simulink model "controladorultimo"  (Simulink 7.9)
settings: Solver=ode45  StartTime=0.0  StopTime=100  RelTol=1e-3
settings Model: Creator=Miguel Faggioni  LastModifiedBy=Miguel Faggioni
settings DataIOCC: TimeSaveName=t

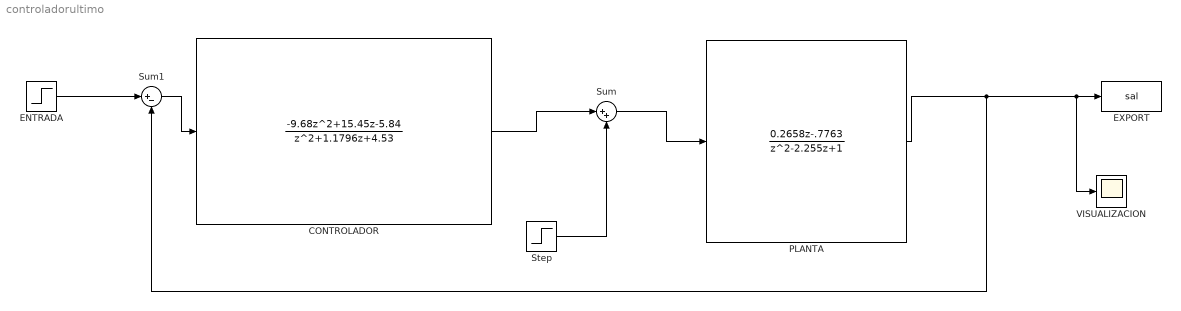
== system controladorultimo ==
  CONTROLADOR : DiscreteTransferFcn  Numerator=[-9.68 15.45 -5.84]  Denominator=[1 1.1796 4.53]
  ENTRADA : Step  Time=0  SampleTime=.5
  EXPORT : ToWorkspace  VariableName=sal  SampleTime=-1
  PLANTA : DiscreteTransferFcn  Numerator=[0.2658 -.7763]  Denominator=[1 -2.255 1]
  Step : Step  SampleTime=.5
  Sum : Sum  Inputs=|++
  Sum1 : Sum  Inputs=|+-
  VISUALIZACION : Scope
      settings: TimeRange=10  YMin=-4e+38  YMax=0
  wires:
  ENTRADA/1 -> Sum1/1
  Sum1/1 -> CONTROLADOR/1
  PLANTA/1 -> Sum1/2, EXPORT/1, VISUALIZACION/1
  CONTROLADOR/1 -> Sum/1
  Sum/1 -> PLANTA/1
  Step/1 -> Sum/2
